simulink model "ExampleSimulinkModel"  (R2018b)
settings: Solver=FixedStepAuto  StartTime=0.0  StopTime=12250  FixedStep=0.05  RelTol=1e-3
settings Model: Creator=Damerius  LastModifiedBy=damerius
settings DebuggingCC: LibraryContextMissingDiagnostic=none
settings SFSimCC: SimUseLocalCustomCode=off
settings RTWCC: RTWUseLocalCustomCode=off

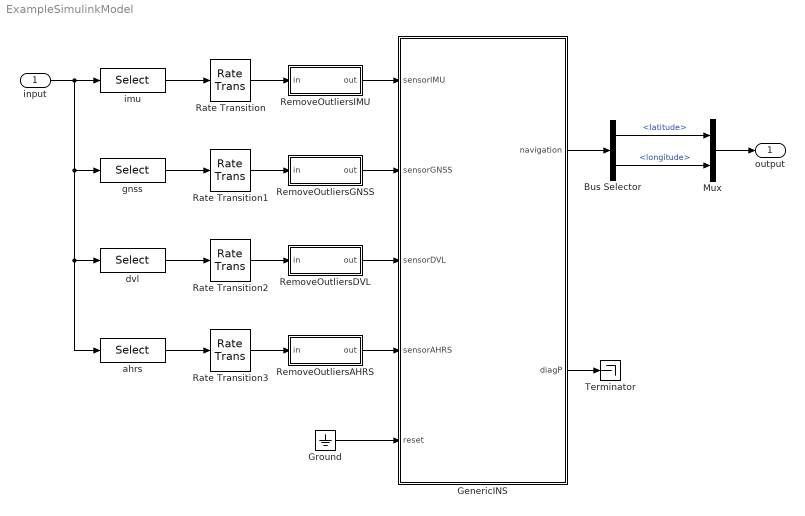
== system ExampleSimulinkModel ==
  input : Inport
  Bus Selector : BusSelector  OutputSignals=latitude,longitude
  GenericINS : Subsystem
  Ground : Ground
  Mux : Mux  Inputs=2
  Rate Transition{,1..3} (4 alike) : RateTransition  Integrity=off  Deterministic=off  OutPortSampleTime=0.05
  RemoveOutliersAHRS : Subsystem
  RemoveOutliersDVL : Subsystem
  RemoveOutliersGNSS : Subsystem
  RemoveOutliersIMU : Subsystem
  Terminator : Terminator
  ahrs : Selector  InputPortWidth=19  IndexOptions=Index vector (dialog)  Indices=16:19  OutputSizes=1
  dvl : Selector  InputPortWidth=19  IndexOptions=Index vector (dialog)  Indices=12:15  OutputSizes=1
  gnss : Selector  InputPortWidth=19  IndexOptions=Index vector (dialog)  Indices=8:11  OutputSizes=1
  imu : Selector  InputPortWidth=19  IndexOptions=Index vector (dialog)  Indices=1:7  OutputSizes=1
  output : Outport
  wires:
  input/1 -> ahrs/1, dvl/1, gnss/1, imu/1
  Mux/1 -> output/1
  Ground/1 -> GenericINS/5(reset)
  Rate Transition1/1 -> RemoveOutliersGNSS/1(in)
  Rate Transition2/1 -> RemoveOutliersDVL/1(in)
  Rate Transition3/1 -> RemoveOutliersAHRS/1(in)
  imu/1 -> Rate Transition/1
  gnss/1 -> Rate Transition1/1
  dvl/1 -> Rate Transition2/1
  ahrs/1 -> Rate Transition3/1
  Rate Transition/1 -> RemoveOutliersIMU/1(in)
  RemoveOutliersIMU/1(out) -> GenericINS/1(sensorIMU)
  RemoveOutliersGNSS/1(out) -> GenericINS/2(sensorGNSS)
  RemoveOutliersDVL/1(out) -> GenericINS/3(sensorDVL)
  RemoveOutliersAHRS/1(out) -> GenericINS/4(sensorAHRS)
  GenericINS/2(diagP) -> Terminator/1
  GenericINS/1(navigation) -> Bus Selector/1
  Bus Selector/2 -> Mux/2  "<longitude>"
  Bus Selector/1 -> Mux/1  "<latitude>"

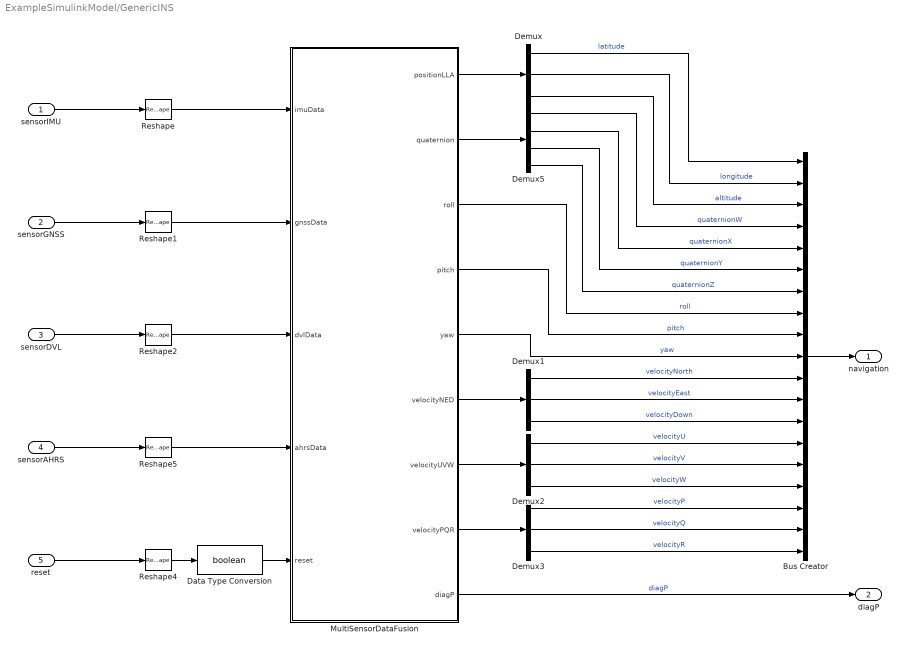
== system ExampleSimulinkModel/GenericINS ==
  sensorIMU : Inport
  sensorGNSS : Inport  Port=2
  sensorDVL : Inport  Port=3
  sensorAHRS : Inport  Port=4
  reset : Inport  Port=5
  Bus Creator : BusCreator  Inputs=19
  Data Type Conversion : DataTypeConversion  OutDataTypeStr=boolean
  Demux{,1..3} (4 alike) : Demux  Outputs=3
  Demux5 : Demux
  MultiSensorDataFusion : MATLAB Function  TreatAsAtomicUnit=on
  Reshape : Reshape  OutputDimensionality=Customize  OutputDimensions=[7,1]
  Reshape1 : Reshape  OutputDimensionality=Customize  OutputDimensions=[4,1]
  Reshape2 : Reshape  OutputDimensionality=Customize  OutputDimensions=[4,1]
  Reshape4 : Reshape  OutputDimensionality=Customize
  Reshape5 : Reshape  OutputDimensionality=Customize  OutputDimensions=[4,1]
  navigation : Outport
  diagP : Outport  Port=2
  wires:
  Reshape5/1 -> MultiSensorDataFusion/4(ahrsData)
  sensorAHRS/1 -> Reshape5/1
  Data Type Conversion/1 -> MultiSensorDataFusion/5(reset)
  reset/1 -> Reshape4/1
  Reshape4/1 -> Data Type Conversion/1
  Reshape2/1 -> MultiSensorDataFusion/3(dvlData)
  Reshape1/1 -> MultiSensorDataFusion/2(gnssData)
  Reshape/1 -> MultiSensorDataFusion/1(imuData)
  sensorGNSS/1 -> Reshape1/1
  sensorDVL/1 -> Reshape2/1
  sensorIMU/1 -> Reshape/1
  MultiSensorDataFusion/1(positionLLA) -> Demux/1
  MultiSensorDataFusion/6(velocityNED) -> Demux1/1
  MultiSensorDataFusion/7(velocityUVW) -> Demux2/1
  MultiSensorDataFusion/8(velocityPQR) -> Demux3/1
  MultiSensorDataFusion/2(quaternion) -> Demux5/1
  Demux/1 -> Bus Creator/1  "latitude"
  Demux/2 -> Bus Creator/2  "longitude"
  Demux/3 -> Bus Creator/3  "altitude"
  Demux5/1 -> Bus Creator/4  "quaternionW"
  Demux5/2 -> Bus Creator/5  "quaternionX"
  Demux5/3 -> Bus Creator/6  "quaternionY"
  Demux5/4 -> Bus Creator/7  "quaternionZ"
  MultiSensorDataFusion/3(roll) -> Bus Creator/8  "roll"
  MultiSensorDataFusion/4(pitch) -> Bus Creator/9  "pitch"
  MultiSensorDataFusion/5(yaw) -> Bus Creator/10  "yaw"
  Demux1/1 -> Bus Creator/11  "velocityNorth"
  Demux1/2 -> Bus Creator/12  "velocityEast"
  Demux1/3 -> Bus Creator/13  "velocityDown"
  Demux2/1 -> Bus Creator/14  "velocityU"
  Demux2/2 -> Bus Creator/15  "velocityV"
  Demux2/3 -> Bus Creator/16  "velocityW"
  Demux3/1 -> Bus Creator/17  "velocityP"
  Demux3/2 -> Bus Creator/18  "velocityQ"
  Demux3/3 -> Bus Creator/19  "velocityR"
  Bus Creator/1 -> navigation/1
  MultiSensorDataFusion/9(diagP) -> diagP/1  "diagP"

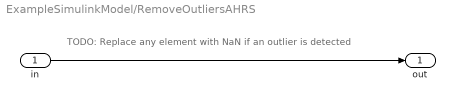
== system ExampleSimulinkModel/RemoveOutliersAHRS ==
  note: TODO: Replace any element with NaN if an outlier is detected
  in : Inport
  out : Outport
  wires:
  in/1 -> out/1

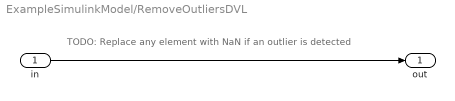
== system ExampleSimulinkModel/RemoveOutliersDVL ==
  note: TODO: Replace any element with NaN if an outlier is detected
  in : Inport
  out : Outport
  wires:
  in/1 -> out/1

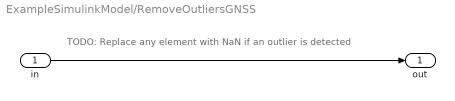
== system ExampleSimulinkModel/RemoveOutliersGNSS ==
  note: TODO: Replace any element with NaN if an outlier is detected
  in : Inport
  out : Outport
  wires:
  in/1 -> out/1

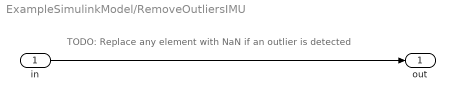
== system ExampleSimulinkModel/RemoveOutliersIMU ==
  note: TODO: Replace any element with NaN if an outlier is detected
  in : Inport
  out : Outport
  wires:
  in/1 -> out/1

== matlab function ExampleSimulinkModel/GenericINS/MultiSensorDataFusion ==
  data: imuData input double size=[7, 1]; gnssData input double size=[4, 1]; positionLLA output double size=[3, 1]; quaternion output double size=[4, 1]; roll output double size=1; pitch output double size=1; yaw output double size=1; velocityNED output double size=[3, 1]; velocityUVW output double size=[3, 1]; velocityPQR output double size=[3, 1]; dvlData input double size=[4, 1]; ahrsData input double size=[4, 1]; reset input boolean size=1; diagP output double size=[12, 1]
function [positionLLA, quaternion, roll, pitch, yaw, velocityNED, velocityUVW, velocityPQR, diagP]  = MultiSensorDataFusion(imuData, gnssData, dvlData, ahrsData, reset)
    persistent genericINS;
    if isempty(genericINS), genericINS = GenericINS(); end

    % Reset filter if required
    if(reset), genericINS.Reset(); end

    % Run step function
    genericINS.Step(imuData, gnssData, dvlData, ahrsData);

    % Get state estimation
    [positionLLA, velocityNED, velocityUVW, velocityPQR, quaternion, roll, pitch, yaw] = genericINS.GetState();
    value = genericINS.GetDiagP();
    diagP = value(1:12);
end
